simulink subsystem "myRMS_fixed"  (R2024a)
settings: Solver=VariableStepAuto  StartTime=0.0  StopTime=10.0  RelTol=1e-3
values from neighbouring files (symbols this model uses):
  a = 1/data(end, 1)    [csv_analize.m]
  b = 1/data(2, 1)    [csv_analize.m]
undefined symbols (not defined in the file or in its folder): BUFFER_LEN, c, SAMPLING_FREQ
libraries: hdlsllib x3, embmathops x1, simulink_extras x1, dspsigops x1
settings Model: Creator=Jan Rosa  LastModifiedBy=Jan Rosa

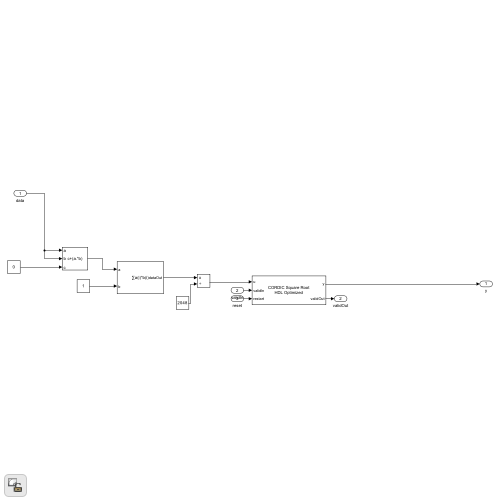
[thumbnail: Simulink's stored preview of the top-level diagram]
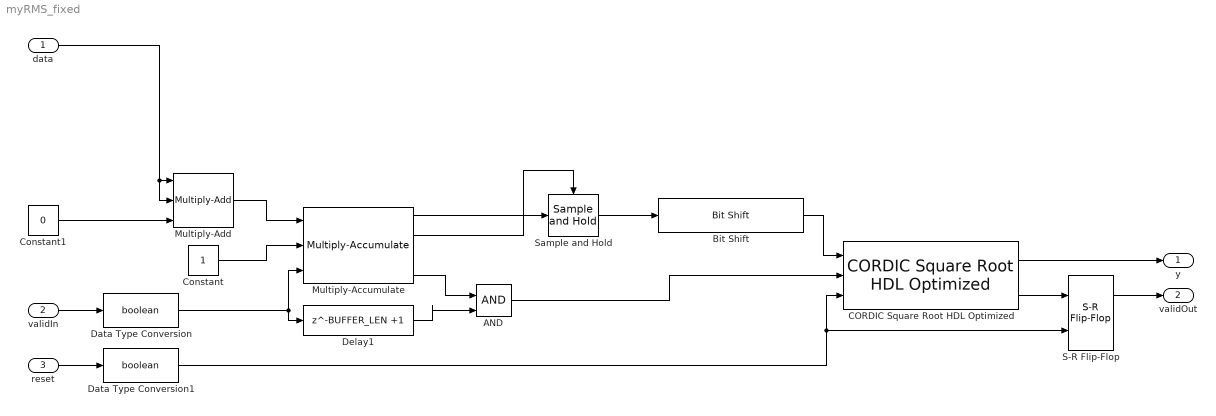
== system myRMS_fixed ==
  data : Inport  OutDataTypeStr=fixdt(1,12,11)
  validIn : Inport  Port=2  OutDataTypeStr=boolean
  reset : Inport  Port=3  OutDataTypeStr=boolean
  AND : Logic  IconShape=distinctive  AllPortsSameDT=off  OutDataTypeStr=boolean
  Bit Shift : hdlsllib/Logic and Bit Operations/Bit Shift  mode=Shift Right Arithmetic  N=log2(BUFFER_LEN)
  CORDIC Square Root HDL Optimized : embmathops/CORDIC Square Root HDL Optimized  autoMaximumShiftVal=on  maximumShiftValue=10  nIterPerReg=1
      settings: LibrarySourceBlock=embeddedMatrixLib/Math Operations/CORDIC Square Root HDL Optimized
  Constant : Constant  OutDataTypeStr=fixdt(0,16,15)  SampleTime=1/SAMPLING_FREQ
  Constant1 : Constant  Value=0  OutDataTypeStr=fixdt(1,12,11)  SampleTime=1/SAMPLING_FREQ
  Data Type Conversion : DataTypeConversion  OutDataTypeStr=boolean  SaturateOnIntegerOverflow=off  RndMeth=Floor
  Data Type Conversion1 : DataTypeConversion  OutDataTypeStr=boolean  SaturateOnIntegerOverflow=off  RndMeth=Floor
  Delay1 : Delay  DelayLength=BUFFER_LEN +1
  Multiply-Accumulate : hdlsllib/HDL Operations/Multiply-Accumulate  opMode=Streaming - using Number of Samples  initValueSetting=Dialog  initValue=0  initValueSetting2=Dialog  initValue2=0  initValueSetting3=Dialog  initValue3=0  num_samples=BUFFER_LEN  RndMeth2=Floor  RndMeth3=Floor  datatype2=Inherit: Inherit via back propagation  datatype3=fixdt(0,16,7)  validOut=on  endInandOut=on  startOut=on  countOut=on  dim=-1  DoSatur=off  parallel=off
  Multiply-Add : hdlsllib/HDL Operations/Multiply-Add  Function=c+(a.*b)  datatype=fixdt(0,16,17)  DoSatur=off  FMA=off
  S-R Flip-Flop : simulink_extras/Flip Flops/S-R Flip-Flop  initial_condition=0
  Sample and Hold : dspsigops/Sample and Hold  trig=Rising edge  initCond=0  latchinput=off
  y : Outport
  validOut : Outport  Port=2
  wires:
  Bit Shift/1 -> CORDIC Square Root HDL Optimized/1
  Multiply-Accumulate/1 -> Sample and Hold/1
  reset/1 -> Data Type Conversion1/1
  data/1 -> Multiply-Add/2, Multiply-Add/1
  Multiply-Add/1 -> Multiply-Accumulate/1
  Constant1/1 -> Multiply-Add/3
  Constant/1 -> Multiply-Accumulate/2
  CORDIC Square Root HDL Optimized/2 -> S-R Flip-Flop/1
  CORDIC Square Root HDL Optimized/1 -> y/1
  validIn/1 -> Data Type Conversion/1
  Sample and Hold/1 -> Bit Shift/1
  Multiply-Accumulate/2 -> Sample and Hold/Trigger
  Data Type Conversion/1 -> Delay1/1, Multiply-Accumulate/3
  Data Type Conversion1/1 -> CORDIC Square Root HDL Optimized/3, S-R Flip-Flop/2
  Multiply-Accumulate/4 -> AND/1
  AND/1 -> CORDIC Square Root HDL Optimized/2
  Delay1/1 -> AND/2
  S-R Flip-Flop/1 -> validOut/1
